simulink model "Model_Vehicle_study_26a"  (R2026a)
settings: Solver=VariableStepAuto  StopTime=300
libraries: fl_lib x7, nesl_utility x4, sdl_lib x3
settings Model: Creator=isaacito  LastModifiedBy=ythvg
settings SimscapeCC: SimscapeNominalValues="[{\"value\":\"1\",\"unit\":\"A\"},{\"value\":\"1\",\"unit\":\"bar\"},{\"value\":\"1\",\"unit\":\"cm^2\"},{\"value\":\"1\",\"unit\":\"cm^3/s\"},{\"value\":\"1\",\"unit\":\"kJ/kg\"},{\"value\":\"1\",\"unit\":\"kW\"},{\"value\":\"1\",\"unit\":\"l\"},{\"value\":\"1\",\"unit\":\"N\"},{\"value\":\"1\",\"unit\":\"N*m\"},{\"value\":\"1\",\"unit\":\"V\"}]"  SimscapeLogSimulationStatistics=on  SimscapeLogLimitData=off  SimscapeLogDataHistory=5000.0

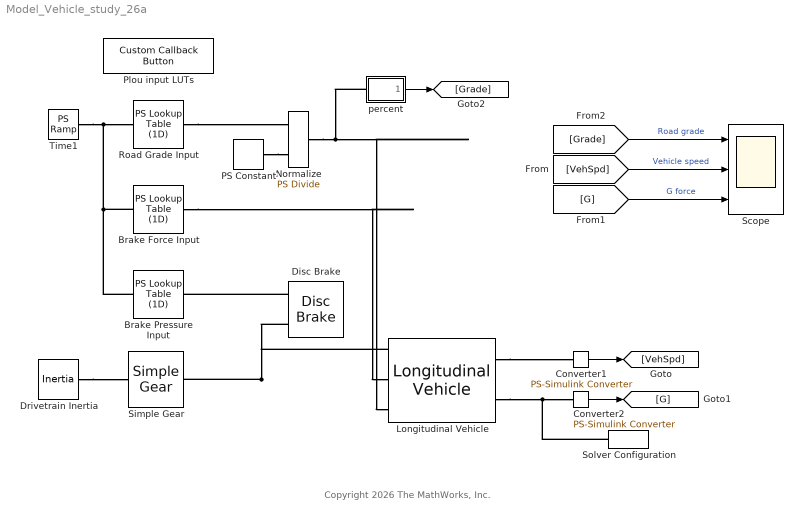
== system Model_Vehicle_study_26a ==
  note: Copyright 2026 The MathWorks, Inc.
  Brake Force Input : fl_lib/Physical Signals/Lookup Tables/PS Lookup Table (1D)  x=[0 1 2] s  f=[0 0 0] N  interp_method=simscape.enum.interpolation.smooth  extrap_method=simscape.enum.extrapolation.nearest
  Brake Pressure Input : fl_lib/Physical Signals/Lookup Tables/PS Lookup Table (1D)  x=[0 1 2] s  f=[0 0 0] Pa  interp_method=simscape.enum.interpolation.smooth  extrap_method=simscape.enum.extrapolation.nearest
  Converter1 : nesl_utility/PS-Simulink Converter  PhysicalDomain=network_engine_domain  SubClassName=ps_output  LeftPortType=input  RightPortType=output  PseudoPeriodic=off  Frequencies=[]  VectorFormat=inherit  Unit=km/hr  AffineConversion=off
  Converter2 : nesl_utility/PS-Simulink Converter  PhysicalDomain=network_engine_domain  SubClassName=ps_output  LeftPortType=input  RightPortType=output  PseudoPeriodic=off  Frequencies=[]  VectorFormat=inherit  Unit=1  AffineConversion=off
  Disc Brake : sdl_lib/Brakes & Detents/Rotational/Disc Brake  r_mean=150 mm  bore=10 mm  n_pads=2  thermal_port=simscape.enum.thermaleffects.omit  mu_static=0.9  mu_coulomb=0.7  temperature_TLU=[280, 300, 320] K  mu_static_TLU=[.9, .8, .7]  mu_coulomb_TLU=[.8, .7, .6]  brkwy_vel=0.1 rad/s  visc_coef=0 N*m*s/rad  thermal_mass=50 kJ/K  temperature_specify=off  temperature_priority=High  temperature=300 K  temperature_nominal_specify=off  temperature_nominal_value=1  temperature_nominal_unit=K
  Drivetrain Inertia : fl_lib/Mechanical/Rotational Elements/Inertia  inertia=20*0.1^2 kg*m^2  num_ports=foundation.enum.numPorts2.one  w_specify=off  w_priority=High  w=0 rad/s  w_nominal_specify=off  w_nominal_value=1  w_nominal_unit=rad/s  t_specify=off  t_priority=None  t=0 N*m  t_nominal_specify=off  t_nominal_value=1  t_nominal_unit=N*m
  Longitudinal Vehicle : sdl_lib/Tires & Vehicles/Longitudinal Vehicle  vehParamType=sdl.enum.VehicleParameterizationType.RoadLoad  M_vehicle=1500 kg  R_tireroll=0.3 m  C_tireroll=0.0136  C_airdrag=0.31  A_front=2.3 m^2  A_rl=120 N  B_rl=0 N*s/m  C_rl=0.03 N*hr^2/km^2  g=9.81 m/s^2  V_1=0.1 m/s  w_1=0.1 rad/s  ShowBrakeIn=true  ShowSlopeIn=true  SlopeInputType=sdl.enum.VehicleLongitudinalRoadSlopeInputType.Grade  ShowWindIn=false  ShowGOut=true  air_density=1.184 kg/m^3  V_x_specify=off  V_x_priority=High  V_x=0 m/s  V_x_nominal_specify=off  V_x_nominal_value=1  V_x_nominal_unit=m/s  trq_specify=off  trq_priority=None  trq=0 N*m  trq_nominal_specify=off  trq_nominal_value=1  trq_nominal_unit=N*m  w_specify=off  w_priority=None  w=0 rad/s  w_nominal_specify=off  w_nominal_value=1  w_nominal_unit=rad/s
  Normalize : fl_lib/Physical Signals/Functions/PS Divide
  PS Constant : fl_lib/Physical Signals/Sources/PS Constant  constant=100
      settings: AttributesFormatString=%<constant>
  Plou input LUTs : CustomCallbackButton  Configuration="{\"components\":[{\"name\":\"BackgroundImageComponent\",\"settings\":{\"image\":{\"size\":[0,0],\"src\":\"default\",\"srcOrientation\":\"Right\"},\"position\":[0,0,1,1]}},{\"name\":\"ButtonStateComponent\",\"settings\":{\"buttonType\":\"momentary\",\"clickFcn\":\"fig = figure;\\nfig.Position(3:4) = [600 700];  % width height\\nModelUtil1.plotLookupTable1DBlocks(gcs, ...\\n  Blocks=[\\n  \\\"Road Grade Input\\\"\\n  \\\"Brake Force Input\\\"\\n  \\\"Brake Pressure Input\\\"\\n  ], ...\\n  ParentAxes=axes(fig))\",\"onValue\":1,\"position\":[0,0,1,1],\"pressDelay\":\"500\",\"pressFcn\":\"\",\"repeatInterval\":\"0\",\"states\":[{\"horizontalAlignment\":\"center\",\"image\":{\"position\":[0,0,1,1],\"size\":[1,1],\"src\":\"default\",\"srcOrientation\":\"Right\"},\"label\":{\"color\":[0.01176470588,0.01176470588,0.01176470588,1],\"icon\":{\"size\":[0,0],\"src\":\"default\",\"srcOrientation\":\"Right\"},\"iconOffset\":0,\"iconPlacement\":\"left\",\"opacity\":1,\"show\":true,\"text\":{\"content\":\"Plot\",\"font\":\"Helvetica\"}},\"labelOffset\":[0,0],\"verticalAlignment\":\"middle\"},{\"horizontalAlignment\":\"center\",\"image\":{\"position\":[0,0,1,1],\"size\":[1,1],\"src\":\"default\",\"srcOrientation\":\"Right\"},\"label\":{\"color\":[0.01176470588,0.01176470588,0.01176470588,1],\"icon\":{\"size\":[0,0],\"src\":\"default\",\"srcOrientation\":\"Right\"},\"iconOffset\":0,\"iconPlacement\":\"left\",\"opacity\":1,\"show\":true,\"text\":{\"content\":\"Plot\",\"font\":\"Helvetica\"}},\"labelOffset\":[0,0],\"verticalAlignment\":\"middle\"},{\"horizontalAlignment\":\"center\",\"image\":{\"position\":[0,0,1,1],\"size\":[1,1],\"src\":\"default\",\"srcOrientation\":\"Right\"},\"label\":{\"color\":[0.01176470588,0.01176470588,0.01176470588,1],\"icon\":{\"size\":[0,0],\"src\":\"default\",\"srcOrientation\":\"Right\"},\"iconOffset\":0,\"iconPlacement\":\"left\",\"opacity\":1,\"show\":true,\"text\":{\"content\":\"Plot\",\"font\":\"Helvetica\"}},\"labelOffset\":[0,0],\"verticalAlignment\":\"middle\"},{\"horizontalAlignment\":\"center\",\"image\":{\"position\":[0,0,1,1],\"size\":[1,1],\"src\":\"default\",\"srcOrientation\":\"Right\"},\"label\":{\"color\":[0.01176470588,0.01176470588,0.01176470588,1],\"icon\":{\"size\":[0,0],\"src\":\"default\",\"srcOrientation\":\"Right\"},\"iconOffset\":0,\"iconPlacement\":\"left\",\"opacity\":1,\"show\":true,\"text\":{\"content\":\"Plot\",\"font\":\"Helvetica\"}},\"labelOffset\":[0,0],\"verticalAlignment\":\"middle\"}]}},{\"name\":\"ForegroundImageComponent\",\"settings\":{\"image\":{\"size\":[0,0],\"src\":\"default\",\"srcOrientation\":\"Right\"},\"isForeground\":1,\"position\":[0,0,1,1]}}],\"derived\":{\"blockParameters\":{\"AutoActivate\":true,\"ButtonText\":\"Plot\",\"ButtonType\":\"Momentary\",\"ClickFcn\":\"fig = figure;\\nfig.Position(3:4) = [600 700];  % width height\\nModelUtil1.plotLookupTable1DBlocks(gcs, ...\\n  Blocks=[\\n  \\\"Road Grade Input\\\"\\n  \\\"Brake Force Input\\\"\\n  \\\"Brake Pressure Input\\\"\\n  ], ...\\n  ParentAxes=axes(fig))\",\"OnValue\":1,\"PressDelay\":\"500\",\"PressFcn\":\"\",\"RepeatInterval\":\"0\",\"fixedAspectRatio\":\"off\"}},\"settings\":{\"BindingType\":\"standalone\",\"autoActivate\":true,\"backgroundColor\":[244,244,244,1],\"backgroundOffset\":0.2,\"backgroundOpacity\":1,\"fixedAspectRatio\":\"off\",\"foregroundColor\":[0.01176470588,0.01176470588,0.01176470588,1],\"migratedFromLegacy\":true,\"useBackgroundColor\":true,\"variant\":\"callback\",\"version\":\"R2025a\"},\"type\":\"Button\"}"  CustomBackgroundColor="{\"color\":[0.9568627451,0.9568627451,0.9568627451],\"show\":true}"
  Road Grade Input : fl_lib/Physical Signals/Lookup Tables/PS Lookup Table (1D)  Description=|  x=[0, 2.5, 5, 10, 25, 40, 80, 85, 90, 110, 130, 165, 200] s  f=[0, 0, 0, -10, -10, -10, 0, 0, 0, 5, 0, 0, 0]  interp_method=simscape.enum.interpolation.smooth  extrap_method=simscape.enum.extrapolation.nearest
      | % This text was automatically inserted by Signal Util.
      | % SignalDesignMatrixStart
      | [0 5 0; 10 40 -10; 80 90 0;
      |  110 nan 5; 130 200 0]
      | 
      | % SignalDesignMatrixEnd
  Scope : Scope  NumInputPorts=3
      settings: ActiveDisplayYMinimum=-11.87456  ActiveDisplayYMaximum=6.87108
  Simple Gear : sdl_lib/Gears/Simple Gear  ratio=1/10  rotation_direction=sdl.enum.shaftOutputDirection.same  friction_model=sdl.enum.gear_efficiencies_load.off  T_noload=0.1 N*m  T_nom=5 N*m  efficiency_nom=0.8  efficiency=0.8  temperature_TLU=[280, 300, 320] K  load_TLU=[1, 5, 10] N*m  efficiency_TLU=[.95, .9, .85]  efficiency_TLU2=[.85, .8, .75; .95, .9, .85; .85, .8, .7]  w_thr=0.01 rad/s  pwr_thr=0.001 W  enable_backlash=false  hardstop_model=simscape.enum.hardstop.smooth  backlash_distance=1e-3 mm  r_base=0.1 m  transition=1e-4 mm  backlash_stiffness=1e6 N/m  backlash_damping=1e3 N*s/m  coeff_rest=0.7  v_tol=0.001 m/s  f_tol=0.001 N  tau=0.1 s  mu_visc=[0, 0] N*m*s/rad  thermal_mass=50 J/K  temperature_specify=off  temperature_priority=High  temperature=300 K  temperature_nominal_specify=off  temperature_nominal_value=1  temperature_nominal_unit=K  x_backlash_specify=off  x_backlash_priority=None  x_backlash=0 mm  x_backlash_nominal_specify=off  x_backlash_nominal_value=1  x_backlash_nominal_unit=mm  f_hardstop_specify=off  f_hardstop_priority=None  f_hardstop=0 N  f_hardstop_nominal_specify=off  f_hardstop_nominal_value=1  f_hardstop_nominal_unit=N  v_backlash_specify=off  v_backlash_priority=None  v_backlash=0 m/s  v_backlash_nominal_specify=off  v_backlash_nominal_value=1  v_backlash_nominal_unit=m/s
      settings: AttributesFormatString=%<ratio>
  Solver Configuration : nesl_utility/Solver Configuration  PhysicalDomain=network_engine_domain  SubClassName=solver  LeftPortType=input  RightPortType=generic  Tones=[]  Harmonics=[]  SimulateNoise=off  Profile=off  UseLocalSampling=off  EnableSwitchedLinearOptims=on  FrequencyDomain=off  UseCCode=off  RelTol=0.001  AbsTol=0.001  MinStep=1e-09  ToWorkspace=off  RevertToSquareIcSolve=off  NumHomotopyIterations=100  PhasorMode=off  PhasorModeNumHarmonics=1  ConsistencySolver=NEWTON_XTOL_AFTER_FTOL  CanonicalOrdering=UNORDERED  OptimizeIntermediates=UNOPTIMIZED  IndexReductionMethod=DerivativeReplacement  DoDC=off  ResidualTolerance=1e-09  ConsistencyTolSource=GLOBAL  ConsistencyAbsTol=0.001  ConsistencyRelTol=0.001  ConsistencyTolFactor=0.001  UseLocalSolver=off  LocalSolverChoice=NE_BACKWARD_EULER_ADVANCER  ResolveIndetEquations=on  FunctionEvalNumThread=1  LocalSolverSampleTime=0.001  DoFixedCost=off  MaxNonlinIter=3  MaxModeIter=2  ComputeImpulses=off  ImpulseIterations=2  LinearAlgebra=auto  LinearAlgebraNumThread=0  EquationFormulation=NE_TIME_EF  DelaysMemoryBudget=1024  AutomaticFiltering=on  FilteringTimeConstant=0.001  PartitionStorageMethod=AS_NEEDED  PartitionMemoryBudget=1024  PartitionMethod=ROBUST  MultibodyUseLocalSolver=off  MultibodyLocalSolverChoice=ODE1  MultibodyLocalSolverSampleTime=0.001
      settings: AttributesFormatString=Local solver: %<UseLocalSolver>
  Time1 : fl_lib/Physical Signals/Sources/PS Ramp  slope=1  start_time=0 s  initial_output=0 s  ZeroCross=true
  percent : Subsystem
  wires:
  [VehSpd] -> Scope/2  "Vehicle speed"
  Converter1/1 -> [VehSpd]
  Converter2/1 -> [G]
  [G] -> Scope/3  "G force"
  [Grade] -> Scope/1  "Road grade"
  percent/1(Out1) -> [Grade]
  connections:
  Solver Configuration/RConn1 -- Longitudinal Vehicle/RConn2 -- Converter2/LConn1
  Time1/RConn1 -- Brake Pressure Input/LConn1 -- Brake Force Input/LConn1 -- Road Grade Input/LConn1
  Drivetrain Inertia/LConn1 -- Simple Gear/LConn1
  Longitudinal Vehicle/RConn1 -- Converter1/LConn1
  Road Grade Input/RConn1 -- Normalize/LConn1
  PS Constant/RConn1 -- Normalize/LConn2
  Normalize/RConn1 -- percent/LConn1 -- Longitudinal Vehicle/LConn3
  Brake Force Input/RConn1 -- Longitudinal Vehicle/LConn2
  Disc Brake/LConn2 -- Simple Gear/RConn1 -- Longitudinal Vehicle/LConn1
  Disc Brake/LConn1 -- Brake Pressure Input/RConn1

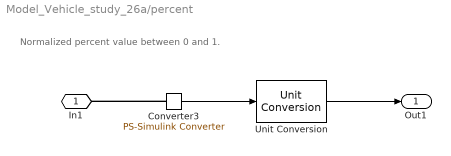
== system Model_Vehicle_study_26a/percent ==
  note: Normalized percent value between 0 and 1.
  Converter3 : nesl_utility/PS-Simulink Converter  PhysicalDomain=network_engine_domain  SubClassName=ps_output  LeftPortType=input  RightPortType=output  PseudoPeriodic=off  Frequencies=[]  VectorFormat=inherit  Unit=1  AffineConversion=off
  Unit Conversion : UnitConversion
  In1 : PMIOPort  Side=Left
  Out1 : Outport  Unit=%
  wires:
  Unit Conversion/1 -> Out1/1
  Converter3/1 -> Unit Conversion/1
  connections:
  Converter3/LConn1 -- In1/RConn1
